simulink library "pv_performance_module"  (R2025b)
settings: Solver=VariableStepAuto  StartTime=0.0  StopTime=10.0  RelTol=1e-3
settings Model: Creator=ciepm  LastModifiedBy=ciepm

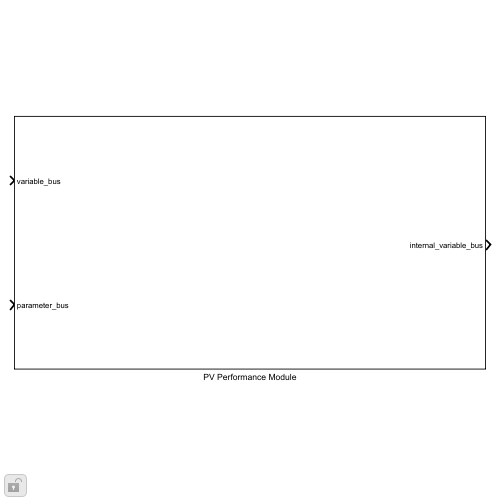
[thumbnail: Simulink's stored preview of the top-level diagram]
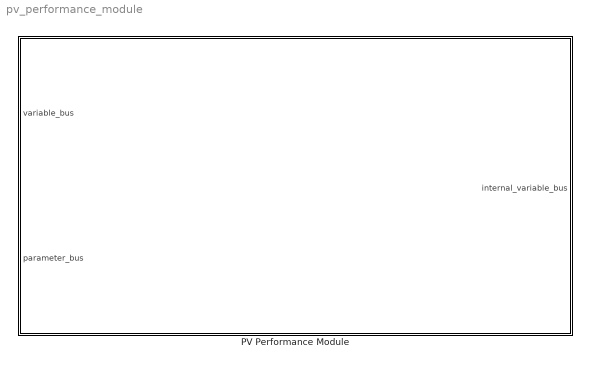
== system pv_performance_module ==
  PV Performance Module : Subsystem

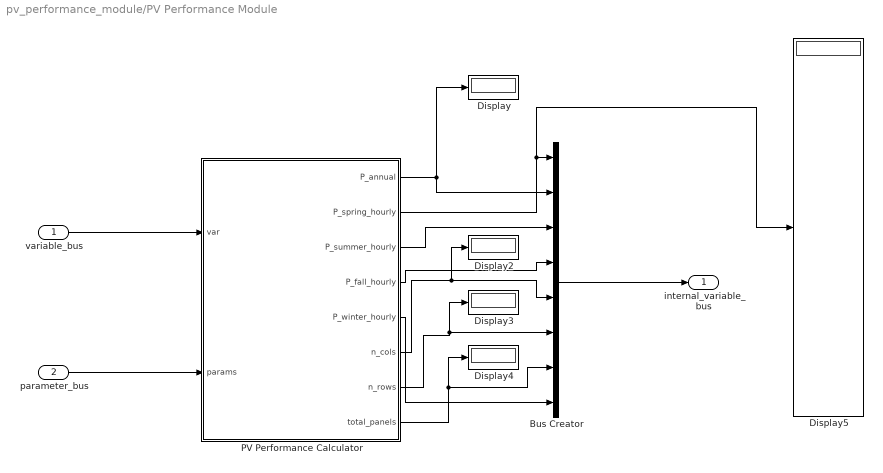
== system pv_performance_module/PV Performance Module ==
  variable_bus : Inport
  parameter_bus : Inport  Port=2
  Bus Creator : BusCreator  Inputs=8
  Display{,2..5} (5 alike) : Display
  PV Performance Calculator : MATLAB Function  TreatAsAtomicUnit=on
  internal_variable_bus : Outport
  wires:
  PV Performance Calculator/5(P_winter_hourly) -> Bus Creator/8
  PV Performance Calculator/8(total_panels) -> Bus Creator/7, Display4/1
  PV Performance Calculator/7(n_rows) -> Display3/1, Bus Creator/6
  PV Performance Calculator/6(n_cols) -> Display2/1, Bus Creator/5
  PV Performance Calculator/1(P_annual) -> Bus Creator/2, Display/1
  variable_bus/1 -> PV Performance Calculator/1(var)
  Bus Creator/1 -> internal_variable_bus/1
  PV Performance Calculator/2(P_spring_hourly) -> Bus Creator/1, Display5/1
  parameter_bus/1 -> PV Performance Calculator/2(params)
  PV Performance Calculator/4(P_fall_hourly) -> Bus Creator/4
  PV Performance Calculator/3(P_summer_hourly) -> Bus Creator/3

== matlab function pv_performance_module/PV Performance Module/PV Performance Calculator ==
  data: var input; P_annual output; params input; P_spring_hourly output; P_summer_hourly output; P_fall_hourly output; P_winter_hourly output; n_cols output; n_rows output; total_panels output
function [P_annual, P_spring_hourly, P_summer_hourly, P_fall_hourly, P_winter_hourly, n_cols, n_rows, total_panels] = pv_model1(var, params)

    %PV model calculating incidence angle, total radiation, and estimated power
    %output
        % DNI ; %direct normal irradiance
        % DHI ; % diffuse horizontal irradiance
        % beta_s ; %sun altitude angle (angle of sun above the local horizon)
        % phi_s ; %sun azimuth angle (angle between the sun and true south)
        l_p = var.PV_l_p; % panel length (m)
        w_p = var.PV_w_p; % panel width (m)
        phi = var.PV_phi; % azimuth angle (radians) - relative to true South, going ccw e.g. pi/2 rad is East
        sigma =var.PV_sigma; % tilt angle (radians) - fixed sloping angle of PV relative to horizontal (xy) plane 
        n_p = params.PV_n_p;%panel efficiency
        x_p = var.PV_x_p; % Distance between panels in a pair/row (m)
        y_p = var.PV_y_p; % Distance between rows (m)
        x = params.land_x; % Total plot width (m)
        y = params.land_y; % Total plot length (m)

    

    %number of panels that fit on the plot
    n_cols = max(1, floor(x / (w_p + x_p)));
    n_rows = max(1, floor(y / (l_p*cos(sigma) + y_p)));
    A_p = l_p*w_p ; %panel area m^2
    
    if n_cols == Inf
        n_cols = 0;
    end
    if n_rows == Inf
        n_rows = 0;
    end
    total_panels = n_rows * n_cols;
    
    [P_spring_daily, P_spring_hourly] = calc_daily_pv(params.weather.spring, phi, sigma, n_p, A_p, total_panels);
    [P_summer_daily, P_summer_hourly] = calc_daily_pv(params.weather.summer, phi, sigma, n_p, A_p, total_panels);
    [P_fall_daily, P_fall_hourly]     = calc_daily_pv(params.weather.fall, phi, sigma, n_p, A_p, total_panels);
    [P_winter_daily, P_winter_hourly] = calc_daily_pv(params.weather.winter, phi, sigma, n_p, A_p, total_panels);
    days_per_season = 365 / 4;
    P_annual = (P_spring_daily + P_summer_daily + P_fall_daily + P_winter_daily) * days_per_season;
    

end
%
function [P_daily, P_hourly] = calc_daily_pv(season_weather, phi, sigma, n_p, A_p, total_panels)
 
    p_tot=0;
    P_hourly = zeros(24,1);
    DNI = season_weather.DNI;
    DHI = season_weather.DHI;
    beta_s = season_weather.beta_s;
    phi_s = season_weather.phi_s;

    for i = 1:24
        if beta_s(i) <= 0
            continue; % Skip to next hour (P_inst remains 0 effectively)
        end
    % Incidence angle
    cos_theta = cos(beta_s(i))*cos(phi_s(i) - phi)*sin(sigma) ...
              + sin(beta_s(i))*cos(sigma);
    
    theta = acos(cos_theta);
    
    % Direct beam
    I_db = DNI(i) .* cos_theta;
    
    % Diffuse irradiance
    I_diff = DHI(i) .* (1 + cos(sigma)) / 2;
    
    % Reflected (Need to double check equation)
    %I_ref = (DNI*sin(beta_s) + DHI) .* albedo .* (1 - cos(tilt)) / 2;
    
    % Total Intercepted Radiation
    R = I_db + I_diff; %+ I_ref;
    
    % Simple power model
    
    p_hour = n_p * A_p * R;          % hourly power per panel
    P_hourly(i) = p_hour*total_panels; % hourly power for entire plot
    p_tot = p_tot + P_hourly(i);
    
    end
    P_daily=p_tot;

    if isnan(P_daily)
        P_daily = 0;
    end
    P_hourly(isnan(P_hourly)) = 0;

end
